simulink model "Water_Heater"  (R2016b)
settings: Solver=ode23t  StartTime=0.0  StopTime=24  RelTol=1e-3  EnableMultiTasking=on
model workspace: external: MAT-File (data not in the file)
settings Model: Creator=jm3gonza  LastModifiedBy=Lenio
settings DataIOCC: SaveFormat=Array  SignalLoggingSaveFormat=ModelDataLogs  SaveOutput=off
settings OptimizationCC: ExpressionDepthLimit=2147483647  LifeSpan=inf
settings DebuggingCC: AlgebraicLoopMsg=none  UnderspecifiedInitializationDetection=Classic  MergeDetectMultiDrivingBlocksExec=none  FcnCallInpInsideContextMsg=warning  UnconnectedInputMsg=none  UnconnectedOutputMsg=none  UnconnectedLineMsg=none  StateNameClashWarn=warning  SFUnexpectedBacktrackingDiag=warning  SFNoUnconditionalDefaultTransitionDiag=warning  SFExecutionAtInitializationDiag=none
settings HardwareCC: ProdBitPerPointer=32  ProdBitPerSizeT=32  ProdBitPerPtrDiffT=32  ProdLargestAtomicFloat=None  ProdIntDivRoundTo=Undefined  ProdEndianess=Unspecified  ProdWordSize=32  ProdHWDeviceType=32-bit Generic
settings ModelReferenceCC: PropagateSignalLabelsOutOfModel=off
settings GRTTargetCC: TargetLangStandard=C89/C90 (ANSI)  GeneratePreprocessorConditionals=Disable all  CombineOutputUpdateFcns=off  GRTInterface=on
settings ConfigComp: CovMetricSettings=dw  CovHtmlReporting=on  CovSaveCumulativeToWorkspaceVar=on  CovSaveSingleToWorkspaceVar=on  CovExternalEMLEnable=off

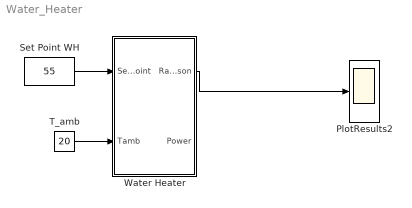
== system Water_Heater ==
  PlotResults2 : Scope
  Set Point WH : Constant  Value=55
  T_amb : Constant  Value=20
  Water Heater : Subsystem
  wires:
  Set Point WH/1 -> Water Heater/1(Set point)
  T_amb/1 -> Water Heater/2(Tamb)
  Water Heater/1(Rate_season) -> PlotResults2/1

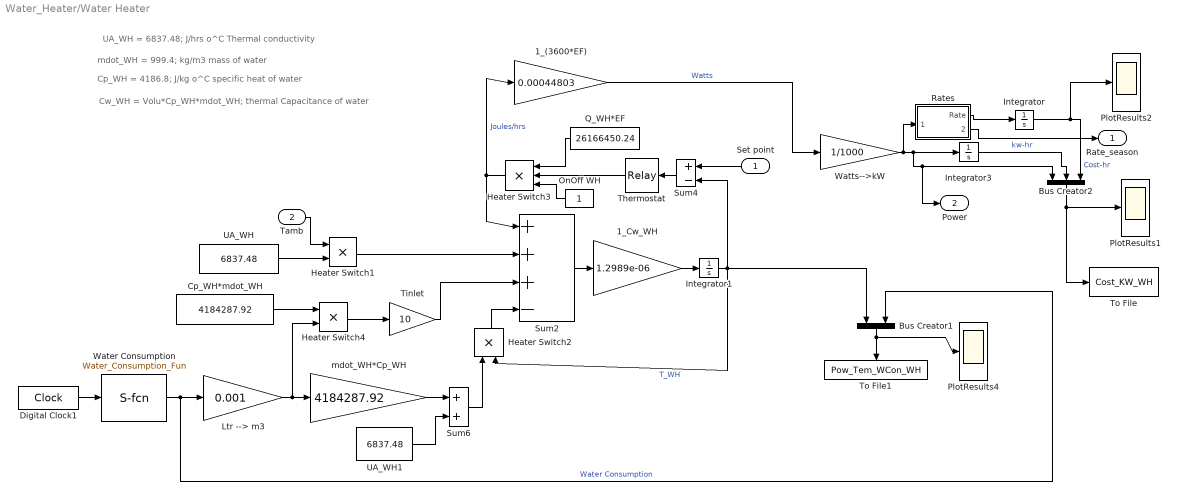
== system Water_Heater/Water Heater ==
  note: UA_WH = 6837.48; J/hrs o^C Thermal conductivity
  note: mdot_WH = 999.4; kg/m3 mass of water
  note: Cp_WH = 4186.8; J/kg o^C specific heat of water
  note: Cw_WH = Volu*Cp_WH*mdot_WH; thermal Capacitance of water
  Set point : Inport
  Tamb : Inport  Port=2
  1_(3600*EF) : Gain  Gain=0.00044803  SaturateOnIntegerOverflow=on  OutDataTypeStr=Inherit: Same as input  ParamDataTypeStr=Inherit: Same as input
  1_Cw_WH : Gain  Gain=1.2989e-06  SaturateOnIntegerOverflow=on  OutDataTypeStr=Inherit: Same as input  ParamDataTypeStr=Inherit: Same as input
  Bus Creator1 : BusCreator  Inputs=2
  Bus Creator2 : BusCreator  Inputs=3
  Cp_WH*mdot_WH : Constant  Value=4184287.92
  Digital Clock1 : DigitalClock
  Heater Switch1 : Product  RndMeth=Zero
  Heater Switch2 : Product  RndMeth=Zero
  Heater Switch3 : Product  Inputs=3  RndMeth=Zero
  Heater Switch4 : Product  RndMeth=Zero
  Integrator : Integrator
  Integrator1 : Integrator  InitialCondition=55
  Integrator3 : Integrator
  Ltr --> m3 : Gain  Gain=0.001
  OnOff WH : Constant  VectorParams1D=off
  PlotResults1 : Scope
  PlotResults2 : Scope
  PlotResults4 : Scope
  Q_WH*EF : Constant  Value=26166450.24  VectorParams1D=off
  Rates : Subsystem
  Sum2 : Sum  Inputs=+++-  SaturateOnIntegerOverflow=on  InputSameDT=on  OutDataTypeStr=Inherit: Same as first input
  Sum4 : Sum  Inputs=+-  SaturateOnIntegerOverflow=on  InputSameDT=on  OutDataTypeStr=Inherit: Same as first input
  Sum6 : Sum  SaturateOnIntegerOverflow=on  InputSameDT=on  OutDataTypeStr=Inherit: Same as first input
  Thermostat : Relay  OnSwitchValue=3  OffSwitchValue=-3
  Tinlet : Gain  Gain=10  SaturateOnIntegerOverflow=on  OutDataTypeStr=Inherit: Same as input  ParamDataTypeStr=Inherit: Same as input
  To File : ToFile  Filename=Cost_KW_WH  MatrixName=Cost_KW_WH
  To File1 : ToFile  Filename=Pow_Tem_WCon_WH  MatrixName=Pow_Tem_WCon_WH
  UA_WH : Constant  Value=6837.48
  UA_WH1 : Constant  Value=6837.48
  Water Consumption : M-S-Function  FunctionName=Water_Consumption_Fun
  Watts-->kW : Gain  Gain=1/1000  SaturateOnIntegerOverflow=on  OutDataTypeStr=Inherit: Same as input  ParamDataTypeStr=Inherit: Same as input
  mdot_WH*Cp_WH : Gain  Gain=4184287.92  SaturateOnIntegerOverflow=on  OutDataTypeStr=Inherit: Same as input  ParamDataTypeStr=Inherit: Same as input
  Rate_season : Outport  InitialOutput=0
  Power : Outport  Port=2  InitialOutput=0
  wires:
  Sum2/1 -> 1_Cw_WH/1
  1_Cw_WH/1 -> Integrator1/1
  Digital Clock1/1 -> Water Consumption/1
  Water Consumption/1 -> Ltr --> m3/1, Bus Creator1/2  "Water Consumption"
  UA_WH/1 -> Heater Switch1/2
  Ltr --> m3/1 -> mdot_WH*Cp_WH/1, Heater Switch4/2
  mdot_WH*Cp_WH/1 -> Sum6/1
  UA_WH1/1 -> Sum6/2
  Sum6/1 -> Heater Switch2/1
  Integrator1/1 -> Heater Switch2/2, Sum4/2, Bus Creator1/1  "T_WH"
  Heater Switch2/1 -> Sum2/4
  Cp_WH*mdot_WH/1 -> Heater Switch4/1
  Heater Switch4/1 -> Tinlet/1
  Tinlet/1 -> Sum2/3
  Heater Switch1/1 -> Sum2/2
  Set point/1 -> Sum4/1
  Sum4/1 -> Thermostat/1
  Q_WH*EF/1 -> Heater Switch3/1
  Heater Switch3/1 -> Sum2/1, 1_(3600*EF)/1  "Joules/hrs"
  1_(3600*EF)/1 -> Watts-->kW/1  "Watts"
  Thermostat/1 -> Heater Switch3/2
  Tamb/1 -> Heater Switch1/1
  Rates/1(Rate) -> Integrator/1
  Watts-->kW/1 -> Rates/1(Powe_cons), Integrator3/1, Bus Creator2/1, Power/1
  Integrator3/1 -> Bus Creator2/2  "kw-hr"
  Bus Creator2/1 -> To File/1, PlotResults1/1
  Bus Creator1/1 -> To File1/1, PlotResults4/1
  Integrator/1 -> PlotResults2/1, Bus Creator2/3  "Cost-hr"
  OnOff WH/1 -> Heater Switch3/3
  Rates/2(Rate_season1) -> Rate_season/1

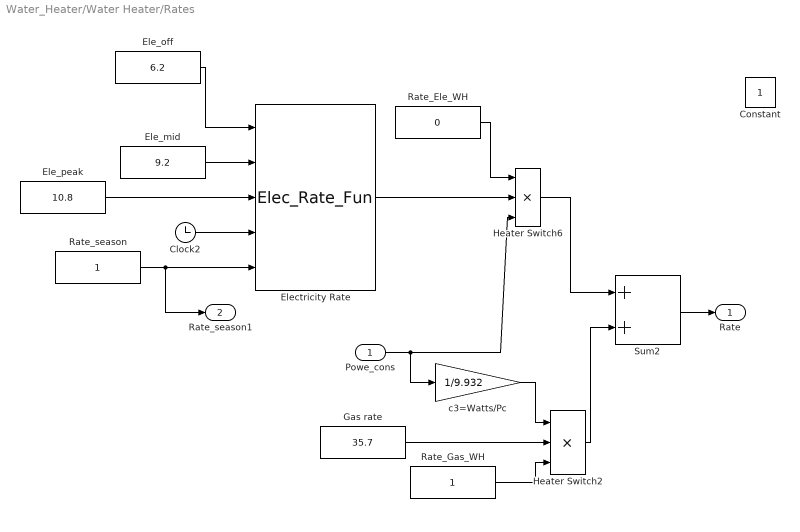
== system Water_Heater/Water Heater/Rates ==
  Powe_cons : Inport
  Clock2 : Clock
      settings: Decimation=100
  Constant : Constant
  Ele_mid : Constant  Value=9.2
  Ele_off : Constant  Value=6.2
  Ele_peak : Constant  Value=10.8
  Electricity Rate : M-S-Function  FunctionName=Elec_Rate_Fun
  Gas rate : Constant  Value=35.7
  Heater Switch2 : Product  Inputs=3  RndMeth=Zero
  Heater Switch6 : Product  Inputs=3  RndMeth=Zero
  Rate_Ele_WH : Constant  Value=0
  Rate_Gas_WH : Constant
  Rate_season : Constant
  Sum2 : Sum  SaturateOnIntegerOverflow=on  InputSameDT=on  OutDataTypeStr=Inherit: Same as first input
  c3=Watts/Pc : Gain  Gain=1/9.932  SaturateOnIntegerOverflow=on  OutDataTypeStr=Inherit: Same as input  ParamDataTypeStr=Inherit: Same as input
  Rate : Outport  InitialOutput=0
  Rate_season1 : Outport  Port=2  InitialOutput=0
  wires:
  Ele_off/1 -> Electricity Rate/1
  Ele_mid/1 -> Electricity Rate/2
  Ele_peak/1 -> Electricity Rate/3
  Clock2/1 -> Electricity Rate/4
  Rate_season/1 -> Electricity Rate/5, Rate_season1/1
  Rate_Ele_WH/1 -> Heater Switch6/1
  Powe_cons/1 -> c3=Watts/Pc/1, Heater Switch6/3
  c3=Watts/Pc/1 -> Heater Switch2/1
  Gas rate/1 -> Heater Switch2/2
  Rate_Gas_WH/1 -> Heater Switch2/3
  Heater Switch6/1 -> Sum2/1
  Heater Switch2/1 -> Sum2/2
  Sum2/1 -> Rate/1
  Electricity Rate/1 -> Heater Switch6/2
